simulink model "DR_Screening_Simulation"  (Simulink 10.0)
settings: Solver=VariableStepDiscrete  StartTime=0.0  StopTime=28800.0  RelTol=1e-3
undefined symbols (not defined in the file or in its folder): cfg
libraries: simeventsqueue1 x4, simeventsserver1 x4, simeventsentitymanagement1 x1, simeventsdelays1 x1, simeventssink1 x1
Description:
  | SIH 2026 AI-Assisted Diabetic Retinopathy Screening Workflow Simulation
  | Member 6: labdhimehta-2311
  | Complete Discrete-Event / Queueing Model: Patient Arrival -> Checkin -> Image Capture -> Network Delay -> AI Inference -> Doctor Review -> Exit

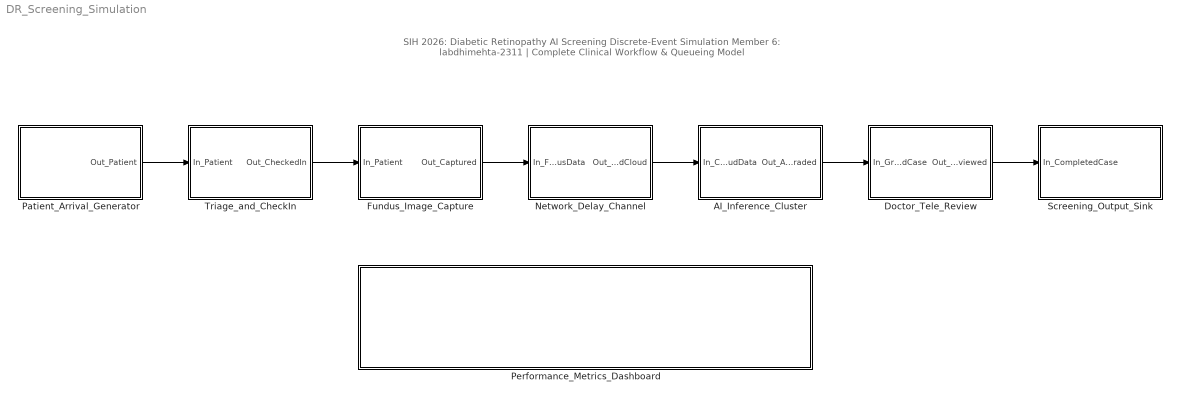
== system DR_Screening_Simulation ==
  note: SIH 2026: Diabetic Retinopathy AI Screening Discrete-Event Simulation
      | Member 6: labdhimehta-2311 | Complete Clinical Workflow & Queueing Model
  Patient_Arrival_Generator : Subsystem
  Triage_and_CheckIn : Subsystem
  Fundus_Image_Capture : Subsystem
  Network_Delay_Channel : Subsystem
  AI_Inference_Cluster : Subsystem
  Doctor_Tele_Review : Subsystem
  Screening_Output_Sink : Subsystem
  Performance_Metrics_Dashboard : Subsystem
  wires:
  Patient_Arrival_Generator/1(Out_Patient) -> Triage_and_CheckIn/1(In_Patient)
  Triage_and_CheckIn/1(Out_CheckedIn) -> Fundus_Image_Capture/1(In_Patient)
  Fundus_Image_Capture/1(Out_Captured) -> Network_Delay_Channel/1(In_FundusData)
  Network_Delay_Channel/1(Out_ArrivedCloud) -> AI_Inference_Cluster/1(In_CloudData)
  AI_Inference_Cluster/1(Out_AIGraded) -> Doctor_Tele_Review/1(In_GradedCase)
  Doctor_Tele_Review/1(Out_Reviewed) -> Screening_Output_Sink/1(In_CompletedCase)

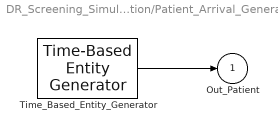
== system DR_Screening_Simulation/Patient_Arrival_Generator ==
  Time_Based_Entity_Generator : simeventsentitymanagement1/Time-Based Entity Generator  distribution=Exponential  mean=3600 / cfg.arrivalRate  entityType=Patient  attributeNames={'PatientID', 'ArrivalTime', 'RiskScore', 'IsHighRisk'}
  Out_Patient : Outport
  wires:
  Time_Based_Entity_Generator/1 -> Out_Patient/1

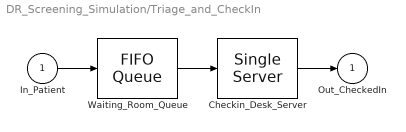
== system DR_Screening_Simulation/Triage_and_CheckIn ==
  In_Patient : Inport
  Waiting_Room_Queue : simeventsqueue1/FIFO Queue  capacity=cfg.patientQueueCapacity
  Checkin_Desk_Server : simeventsserver1/Single Server  servicePeriod=cfg.checkinTime
  Out_CheckedIn : Outport
  wires:
  In_Patient/1 -> Waiting_Room_Queue/1
  Waiting_Room_Queue/1 -> Checkin_Desk_Server/1
  Checkin_Desk_Server/1 -> Out_CheckedIn/1

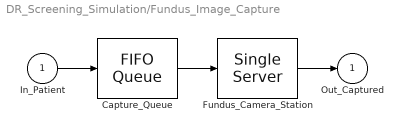
== system DR_Screening_Simulation/Fundus_Image_Capture ==
  In_Patient : Inport
  Capture_Queue : simeventsqueue1/FIFO Queue
  Fundus_Camera_Station : simeventsserver1/Single Server  servicePeriod=cfg.imageCaptureTime
  Out_Captured : Outport
  wires:
  In_Patient/1 -> Capture_Queue/1
  Capture_Queue/1 -> Fundus_Camera_Station/1
  Fundus_Camera_Station/1 -> Out_Captured/1

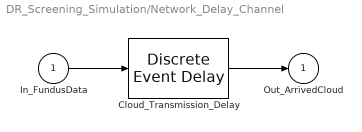
== system DR_Screening_Simulation/Network_Delay_Channel ==
  In_FundusData : Inport
  Cloud_Transmission_Delay : simeventsdelays1/Discrete Event Delay  delayTime=cfg.networkDelay / 1000
  Out_ArrivedCloud : Outport
  wires:
  In_FundusData/1 -> Cloud_Transmission_Delay/1
  Cloud_Transmission_Delay/1 -> Out_ArrivedCloud/1

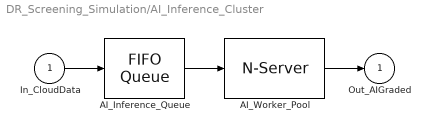
== system DR_Screening_Simulation/AI_Inference_Cluster ==
  In_CloudData : Inport
  AI_Inference_Queue : simeventsqueue1/FIFO Queue
  AI_Worker_Pool : simeventsserver1/N-Server  numberOfServers=cfg.numberOfAIWorkers  servicePeriod=cfg.aiProcessingTime
  Out_AIGraded : Outport
  wires:
  In_CloudData/1 -> AI_Inference_Queue/1
  AI_Inference_Queue/1 -> AI_Worker_Pool/1
  AI_Worker_Pool/1 -> Out_AIGraded/1

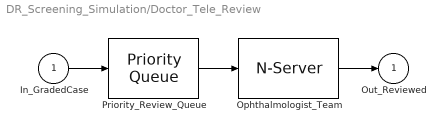
== system DR_Screening_Simulation/Doctor_Tele_Review ==
  In_GradedCase : Inport
  Priority_Review_Queue : simeventsqueue1/Priority Queue  sortingAttribute='IsHighRisk'  sortingDirection=Descending
  Ophthalmologist_Team : simeventsserver1/N-Server  numberOfServers=cfg.numberOfDoctors  servicePeriod=cfg.doctorReviewTime
  Out_Reviewed : Outport
  wires:
  In_GradedCase/1 -> Priority_Review_Queue/1
  Priority_Review_Queue/1 -> Ophthalmologist_Team/1
  Ophthalmologist_Team/1 -> Out_Reviewed/1

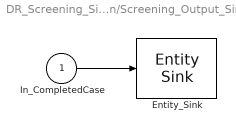
== system DR_Screening_Simulation/Screening_Output_Sink ==
  In_CompletedCase : Inport
  Entity_Sink : simeventssink1/Entity Sink
  wires:
  In_CompletedCase/1 -> Entity_Sink/1

== system DR_Screening_Simulation/Performance_Metrics_Dashboard ==
  note: Real-Time Queue Observers & Little's Law Verifier
      | Monitors Queues, Latency Distributions, and Station Utilizations
